simulink model "soccer_vision"  (R2018b)
settings: Solver=FixedStepAuto  StartTime=0.0  StopTime=inf  FixedStep=0.1  RelTol=1e-3
PreLoadFcn:
  | addpath('soccer-vision/media')
  | addpath('soccer-vision/vectormath')
  | 
  | soccer_vision_parameters
InitFcn:
  | soccer_vision_parameters
values from neighbouring files (symbols this model uses):
  imageHeight = 240    [soccer_vision_parameters.m]
  imageWidth = 320    [soccer_vision_parameters.m]
  sampleTime = 1/30    (= 0.0333333333333)    [soccer_vision_parameters.m]
undefined symbols (not defined in the file or in its folder): focal_length, gray, Pose, Rec, SDTV
libraries: robotlib x6, robotcorelib x2, visiontextngfix x2, visiontransforms x2, dspindex x2, simulink_extras x1, visionanalysis x1, visionstatistics x1, visionconversions x1, dspvision x1
settings Model: NumberOfSteps=100  Creator=vuwij  LastModifiedBy=common
settings OptimizationCC: EnhancedBackFolding=on  PassReuseOutputArgsAs=Individual arguments  MaxStackSize=64  OptimizeBlockOrder=speed  DifferentSizesBufferReuse=on  OptimizationCustomize=off
settings DebuggingCC: ParameterTunabilityLossMsg=error  LibraryContextMissingDiagnostic=none
settings HardwareCC: ProdBitPerLong=64  ProdLargestAtomicInteger=Long  ProdLargestAtomicFloat=Double  ProdLongLongMode=on  ProdHWDeviceType=ARM Compatible->ARM 64-bit (LP64)  TargetHWDeviceType=Generic->Unspecified (assume 32-bit Generic)
settings SFSimCC: SimUseLocalCustomCode=off  MATLABDynamicMemAlloc=off
settings RTWCC: SystemTargetFile=ert.tlc  HardwareBoard=Robot Operating System (ROS)  TLCOptions="-aInlineSetEventsForThisBaseRateFcn=TLC_FALSE -aSuppressMultiTaskScheduler=TLC_FALSE  -aRateBasedStepFcn=0"  TemplateMakefile=ert_default_tmf  GenerateReport=on  RTWUseLocalCustomCode=off  Toolchain=Catkin  IncludeHyperlinkInReport=on  LaunchReport=on  PortableWordSizes=on  TargetLang=C++  GenerateTraceInfo=on  GenerateTraceReport=on  GenerateTraceReportSl=on  GenerateTraceReportSf=on  GenerateTraceReportEml=on
settings CodeAppCC: ForceParamTrailComments=on  IgnoreCustomStorageClasses=off  MaxIdLength=95  OperatorAnnotations=on  SimulinkDataObjDesc=on  SFDataObjDesc=on  InsertBlockDesc=on
settings ERTTargetCC: MultiInstanceERTCode=on  CodeInterfacePackaging=C++ class  SupportVariableSizeSignals=on  RootIOFormat=Structure reference

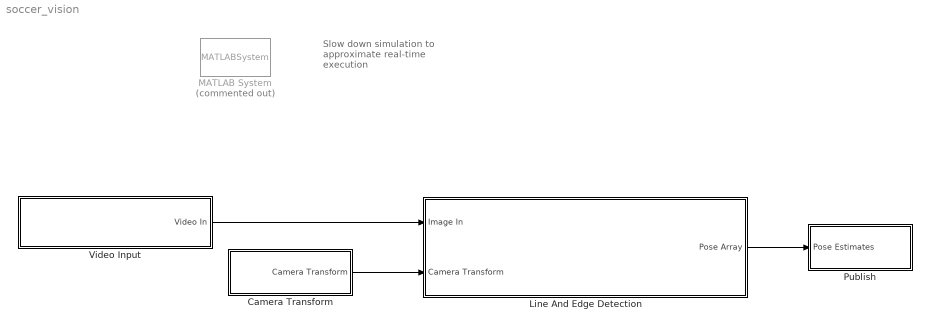
== system soccer_vision ==
  note: Slow down simulation to approximate real-time execution
  Camera Transform : Subsystem  Variant=on
  Line And Edge Detection : Subsystem
  MATLAB System : MATLABSystem  Commented=on  System=ExampleHelperSimulationRateControl  SampleTime=sampleTime
      mask Type: ExampleHelperSimulationRateControl
      mask Display: disp('Rate Control');
  Publish : Subsystem  Variant=on
  Video Input : Subsystem  Variant=on
  wires:
  Video Input/1(Video In) -> Line And Edge Detection/1(Image In)
  Camera Transform/1(Camera Transform) -> Line And Edge Detection/2(Camera Transform)
  Line And Edge Detection/1(Pose Array) -> Publish/1(Pose Estimates)

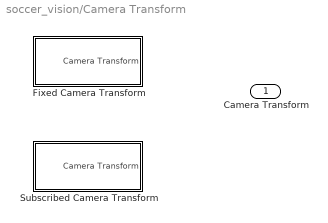
== system soccer_vision/Camera Transform ==
  Fixed Camera Transform : Subsystem  VariantControl=VSS_VIDEO_INPUT
  Subscribed Camera Transform : Subsystem  VariantControl=(default)
  Camera Transform : Outport

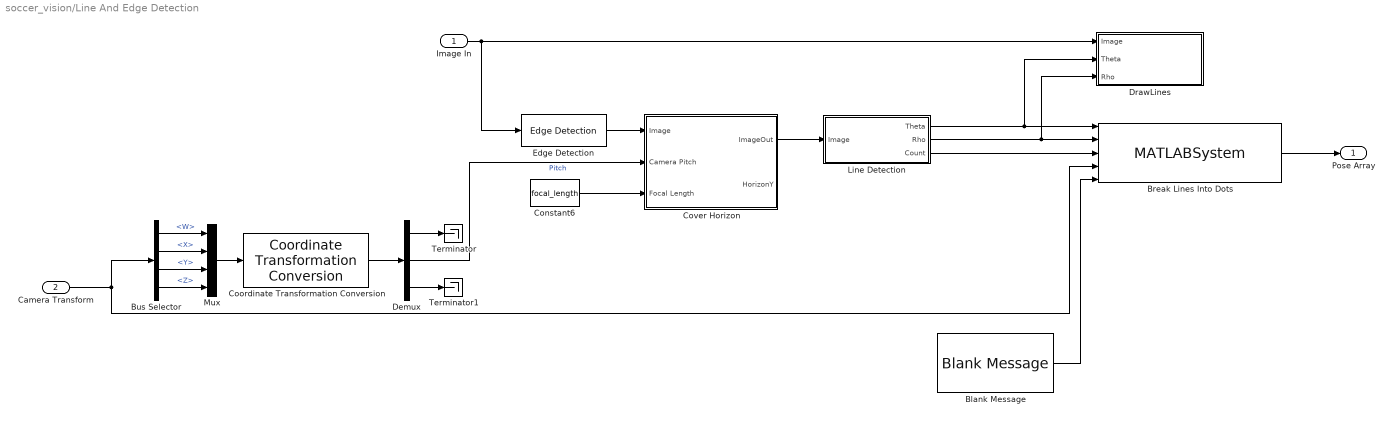
== system soccer_vision/Line And Edge Detection ==
  Image In : Inport  OutDataTypeStr=uint8  PortDimensions=[240 320]  SampleTime=[0.1,0]
  Camera Transform : Inport  Port=2  PortDimensions=1
  Blank Message : robotlib/Blank Message  messageClass=Message  entityType=geometry_msgs/PoseArray  messageType=geometry_msgs/PoseArray  SampleTime=inf
      settings: SourceProductBaseCode=RO
  Break Lines Into Dots : MATLABSystem  System=BreakLinesIntoDots  width=360  height=240  init_pitch=30  init_height=0.5  SimulateUsing=Interpreted execution
      mask Type: BreakLinesIntoDots
      mask Display:
      | disp('BreakLinesIntoDots');
      | port_label('input',1,'thetas');
      | port_label('input',2,'rhos');
      | port_label('input',3,'counts');
      | port_label('input',4,'camerapose');
      | port_label('input',5,'posearray');
      | port_label('output',1,'posearray');
  Bus Selector : BusSelector  OutputSignals=Pose.Orientation.W,Pose.Orientation.X,Pose.Orientation.Y,Pose.Orientation.Z
  Constant6 : Constant  Value=focal_length
  Coordinate Transformation Conversion : robotcorelib/Coordinate Transformation Conversion  InputRepresentation=Quaternion  InputEulerSequence=ZYX  ShowTrVecInputPort=on  OutputRepresentation=Euler Angles  OutputEulerSequence=XYZ  ShowTrVecOutputPort=on  SimulateUsing=Code generation
      settings: SourceProductBaseCode=RO
  Cover Horizon : Subsystem
  Demux : Demux  Outputs=3
  DrawLines : Subsystem
  Edge Detection : visionanalysis/Edge Detection  method=Roberts  outputType=Binary image  userDefinedThreshold=off  thresholdSource=Input port  threshold=20  thresholdTuning=9  edgeThinning=off  threshold_canny=[0.25 0.60]  autoPercent=70  sigma=1  roundingMode=Floor  overflowMode=off  prodOutputMode=Binary point scaling  prodOutputWordLength=32  prodOutputFracLength=8  prodOutputSlope=2^-8  accumSlope=2^-8  outputSlope=2^-4
      settings: SourceProductName=Computer Vision System Toolbox  SourceProductBaseCode=VP
  Line Detection : Subsystem
  Mux : Mux
  Terminator : Terminator
  Terminator1 : Terminator
  Pose Array : Outport
  wires:
  Constant6/1 -> Cover Horizon/3("Focal Length ")
  Demux/2 -> Cover Horizon/2(Camera Pitch)  "Pitch"
  Image In/1 -> Edge Detection/1, DrawLines/1(Image)
  Cover Horizon/1(ImageOut) -> Line Detection/1(Image)
  Edge Detection/1 -> Cover Horizon/1(Image)
  Line Detection/1(Theta) -> DrawLines/2(Theta), Break Lines Into Dots/1
  Line Detection/2(Rho) -> Break Lines Into Dots/2, DrawLines/3(Rho)
  Break Lines Into Dots/1 -> Pose Array/1
  Line Detection/3(Count) -> Break Lines Into Dots/3
  Bus Selector/1 -> Mux/1  "<W>"
  Demux/3 -> Terminator1/1
  Camera Transform/1 -> Break Lines Into Dots/4, Bus Selector/1
  Bus Selector/3 -> Mux/3  "<Y>"
  Demux/1 -> Terminator/1
  Bus Selector/4 -> Mux/4  "<Z>"
  Bus Selector/2 -> Mux/2  "<X>"
  Coordinate Transformation Conversion/1 -> Demux/1
  Mux/1 -> Coordinate Transformation Conversion/1
  Blank Message/1 -> Break Lines Into Dots/5

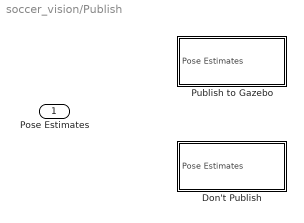
== system soccer_vision/Publish ==
  Pose Estimates : Inport
  Don't Publish : Subsystem  VariantControl=VSS_VIDEO_INPUT
  Publish to Gazebo : Subsystem  VariantControl=(default)

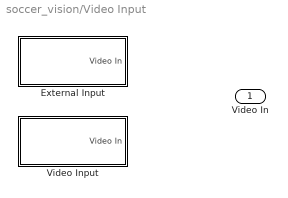
== system soccer_vision/Video Input ==
  External Input : Subsystem  VariantControl=(default)
  Video Input : Subsystem  VariantControl=VSS_VIDEO_INPUT
  Video In : Outport

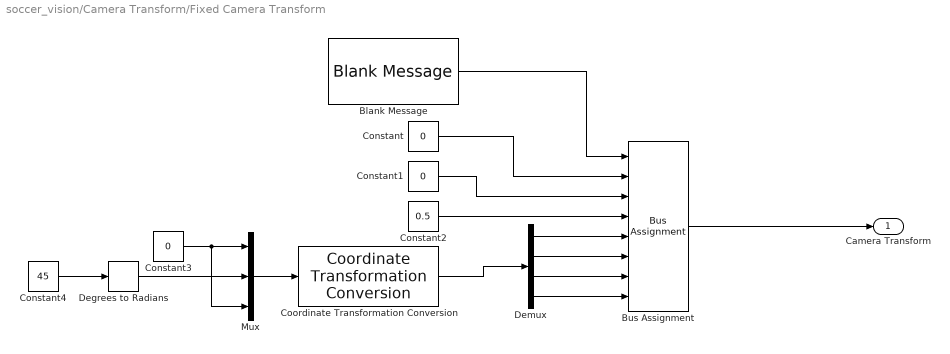
== system soccer_vision/Camera Transform/Fixed Camera Transform ==
  Blank Message : robotlib/Blank Message  messageClass=Message  entityType=geometry_msgs/PoseStamped  messageType=geometry_msgs/PoseStamped  SampleTime=inf
      settings: SourceProductBaseCode=RO
  Bus Assignment : BusAssignment  AssignedSignals=Pose.Position.X,Pose.Position.Y,Pose.Position.Z,Pose.Orientation.X,Pose.Orientation.Y,Pose.Orientation.Z,Pose.Orientation.W
  Constant : Constant  Value=0
  Constant1 : Constant  Value=0
  Constant2 : Constant  Value=0.5
  Constant3 : Constant  Value=0
  Constant4 : Constant  Value=45
  Coordinate Transformation Conversion : robotcorelib/Coordinate Transformation Conversion  InputRepresentation=Euler Angles  InputEulerSequence=ZYX  ShowTrVecInputPort=on  OutputRepresentation=Quaternion  OutputEulerSequence=ZYX  ShowTrVecOutputPort=on  SimulateUsing=Code generation
      settings: SourceProductBaseCode=RO
  Degrees to Radians : simulink_extras/Transformations/Degrees to Radians
  Demux : Demux
  Mux : Mux  Inputs=3
  Camera Transform : Outport
  wires:
  Constant/1 -> Bus Assignment/2
  Blank Message/1 -> Bus Assignment/1
  Bus Assignment/1 -> Camera Transform/1
  Constant1/1 -> Bus Assignment/3
  Constant2/1 -> Bus Assignment/4
  Demux/1 -> Bus Assignment/5
  Demux/2 -> Bus Assignment/6
  Demux/3 -> Bus Assignment/7
  Demux/4 -> Bus Assignment/8
  Coordinate Transformation Conversion/1 -> Demux/1
  Mux/1 -> Coordinate Transformation Conversion/1
  Constant3/1 -> Mux/3, Mux/1
  Degrees to Radians/1 -> Mux/2
  Constant4/1 -> Degrees to Radians/1

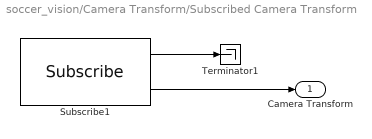
== system soccer_vision/Camera Transform/Subscribed Camera Transform ==
  Subscribe1 : robotlib/Subscribe  topicSource=Specify your own  topic=/soccerbot/poses/camera  messageType=geometry_msgs/Pose  sampleTime=-1  messageQueueLength=1
      settings: SourceProductBaseCode=RO
  Terminator1 : Terminator
  Camera Transform : Outport
  wires:
  Subscribe1/1 -> Terminator1/1
  Subscribe1/2 -> Camera Transform/1

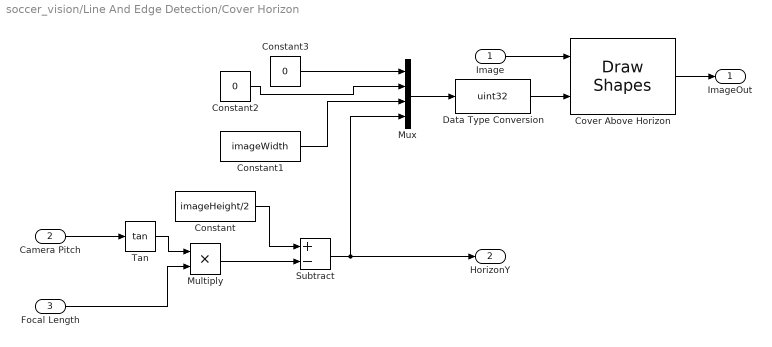
== system soccer_vision/Line And Edge Detection/Cover Horizon ==
  Image : Inport
  Camera Pitch : Inport  Port=2
  "Focal Length " : Inport  Port=3
  Constant : Constant  Value=imageHeight/2
  Constant1 : Constant  Value=imageWidth
  Constant2 : Constant  Value=0
  Constant3 : Constant  Value=0
  Cover Above Horizon : visiontextngfix/Draw Shapes  shape=Rectangles  fill=on  lineWidth=1  fillClrSource=Specify via dialog  display=Black  intensity=200  color=[255 0 0]  opacity=1  viewport=Entire image  antialiasing=off  inType=Obsolete  imagePorts=One multidimensional signal  prodOutputMode=Binary point scaling  prodOutputWordLength=32  prodOutputFracLength=14  memoryMode=Specify word length  memoryWordLength=16  memoryFracLength=14  roundingMode=Floor  overflowMode=off
      settings: SourceProductName=Computer Vision System Toolbox
  Data Type Conversion : DataTypeConversion  OutDataTypeStr=uint32
  Multiply : Product
  Mux : Mux
  Subtract : Sum  Inputs=+-
  Tan : Trigonometry  Operator=tan
  ImageOut : Outport
  HorizonY : Outport  Port=2
  wires:
  Camera Pitch/1 -> Tan/1
  Tan/1 -> Multiply/1
  "Focal Length "/1 -> Multiply/2
  Constant/1 -> Subtract/1
  Multiply/1 -> Subtract/2
  Mux/1 -> Data Type Conversion/1
  Constant3/1 -> Mux/1
  Constant2/1 -> Mux/2
  Constant1/1 -> Mux/3
  Subtract/1 -> Mux/4, HorizonY/1
  Image/1 -> Cover Above Horizon/1
  Data Type Conversion/1 -> Cover Above Horizon/2
  Cover Above Horizon/1 -> ImageOut/1

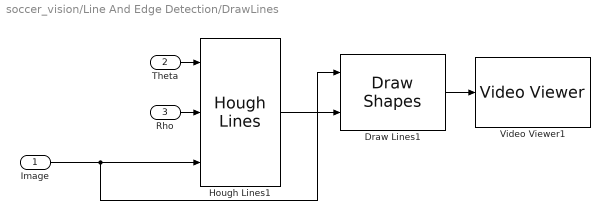
== system soccer_vision/Line And Edge Detection/DrawLines ==
  Image : Inport
  Theta : Inport  Port=2
  Rho : Inport  Port=3
  Draw Lines1 : visiontextngfix/Draw Shapes  shape=Lines  fill=off  lineWidth=1  fillClrSource=Specify via dialog  display=White  intensity=200  color=[255 0 0]  opacity=0.6  viewport=Entire image  antialiasing=off  inType=Obsolete  imagePorts=One multidimensional signal  prodOutputMode=Binary point scaling  prodOutputWordLength=32  prodOutputFracLength=14  memoryMode=Specify word length  memoryWordLength=16  memoryFracLength=14  roundingMode=Floor  overflowMode=off
      settings: SourceProductName=Computer Vision System Toolbox
  Hough Lines1 : visiontransforms/Hough Lines  sineCompMethod=Trigonometric function  thetaRes=pi/180  firstCoeffMode=Specify word length  firstCoeffWordLength=16  firstCoeffFracLength=15  prodOutputMode=Binary point scaling  prodOutputWordLength=32  prodOutputFracLength=16  roundingMode=Nearest  overflowMode=on
      settings: SourceProductName=Computer Vision System Toolbox  SourceProductBaseCode=VP
  Video Viewer1 : VideoViewer  colormapValue=gray(256)  FigPos=[297 924 1134 598]
  wires:
  Theta/1 -> Hough Lines1/1
  Draw Lines1/1 -> Video Viewer1/1
  Hough Lines1/1 -> Draw Lines1/2
  Image/1 -> Draw Lines1/1, Hough Lines1/3
  Rho/1 -> Hough Lines1/2

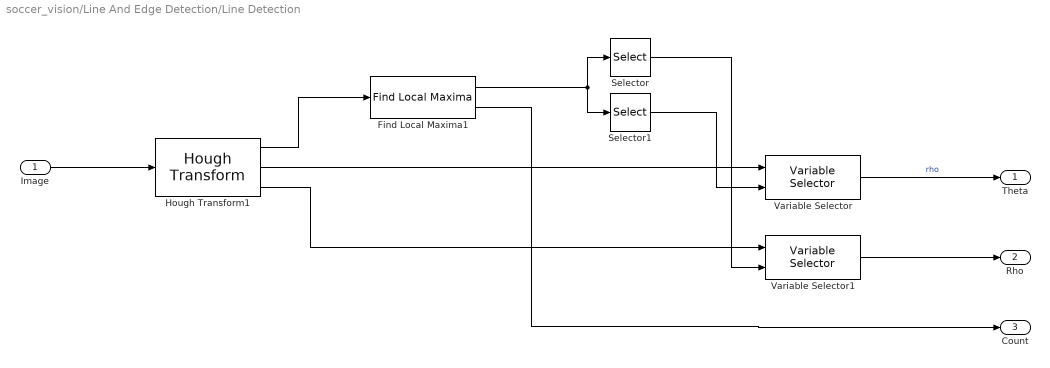
== system soccer_vision/Line And Edge Detection/Line Detection ==
  Image : Inport
  Find Local Maxima1 : visionstatistics/Find Local Maxima  num_peaks=3  nhood_size=[201 41]  src_thresh=Obsolete9b  src_thresh_inuse=Specify via dialog  threshold=100  inputIsHough=on  dt_peak=uint32  isOutVarDim=off  dt_count=uint32
      settings: SourceProductName=Computer Vision System Toolbox  SourceProductBaseCode=VP
  Hough Transform1 : visiontransforms/Hough Transform  theta_res=pi/180  rho_res=1  out_theta_rho=on  outdtmode=double  roundingMode=Nearest  overflowMode=on  firstCoeffMode=Binary point scaling  firstCoeffWordLength=16  firstCoeffFracLength=14  firstCoeffSlope=2^-14  secondCoeffMode=Binary point scaling  secondCoeffWordLength=32  secondCoeffFracLength=16  secondCoeffSlope=2^-16  prodOutputMode=Binary point scaling  prodOutputWordLength=32  prodOutputFracLength=20  prodOutputSlope=2^-20  accumMode=Binary point scaling  accumWordLength=32  accumFracLength=20  accumSlope=2^-20  outputMode=Binary point scaling  outputWordLength=16  outputFracLength=0  outputSlope=2^0  memoryMode=Binary point scaling  memoryWordLength=32  memoryFracLength=16  memorySlope=2^-16
      settings: SourceProductName=Computer Vision System Toolbox  SourceProductBaseCode=VP
  Selector : Selector  NumberOfDimensions=2  InputPortWidth=2  IndexOptions=Select all,Index vector (dialog)  Indices=1,2  OutputSizes=1,1
  Selector1 : Selector  NumberOfDimensions=2  InputPortWidth=2  IndexOptions=Select all,Index vector (dialog)  Indices=0,1  OutputSizes=1,1
  Variable Selector : dspindex/Variable Selector  NumInputs=1  rowsOrCols=Columns  IdxMode=Variable  Elements=[1 3]  ZerOneIdxMode=One-based  errmode=Clip Index  FillMode=on  FillValues=0
  Variable Selector1 : dspindex/Variable Selector  NumInputs=1  rowsOrCols=Columns  IdxMode=Variable  Elements=[1 3]  ZerOneIdxMode=One-based  errmode=Clip Index  FillMode=on  FillValues=0
  Theta : Outport
  Rho : Outport  Port=2
  Count : Outport  Port=3
  wires:
  Hough Transform1/3 -> Variable Selector1/1
  Image/1 -> Hough Transform1/1
  Variable Selector1/1 -> Rho/1
  Variable Selector/1 -> Theta/1  "rho"
  Selector1/1 -> Variable Selector/2
  Selector/1 -> Variable Selector1/2
  Find Local Maxima1/1 -> Selector/1, Selector1/1
  Hough Transform1/2 -> Variable Selector/1
  Hough Transform1/1 -> Find Local Maxima1/1
  Find Local Maxima1/2 -> Count/1

== system soccer_vision/Publish/Don't Publish ==
  Pose Estimates : Inport
  Terminator : Terminator
  wires:
  Pose Estimates/1 -> Terminator/1

== system soccer_vision/Publish/Publish to Gazebo ==
  Pose Estimates : Inport
  Publish : robotlib/Publish  topicSource=Specify your own  topic=/soccerbot/vision_poses  messageType=geometry_msgs/PoseArray  messageQueueLength=1
      settings: SourceProductBaseCode=RO
  wires:
  Pose Estimates/1 -> Publish/1

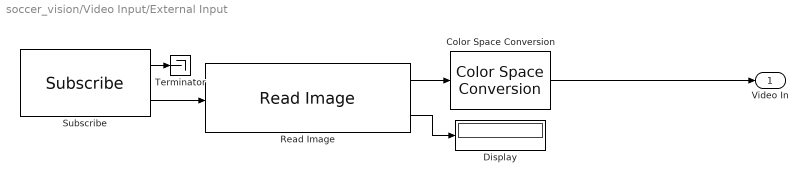
== system soccer_vision/Video Input/External Input ==
  Color Space Conversion : visionconversions/Color Space  Conversion  conversion=Obsolete  conversionActive=R'G'B' to intensity  wp_str=D65  rec=Rec. 601 (SDTV)  sys=1125/60/2:1  imagePorts=One multidimensional signal
      settings: SourceProductName=Computer Vision System Toolbox
  Display : Display
  Read Image : robotlib/Read Image  MaximumImageSize=[240, 320]  ImageEncoding=rgb8  ShowAlphaOutput=off  ShowErrorCodeOutput=on  VariableSizeOutputs=off
      settings: SourceProductName=Robotics System Toolbox  SourceProductBaseCode=RO
  Subscribe : robotlib/Subscribe  topicSource=Select from ROS network  topic=/soccerbot/camera1/image_raw  messageType=sensor_msgs/Image  sampleTime=-1  messageQueueLength=1
      settings: SourceProductBaseCode=RO
  Terminator : Terminator
  Video In : Outport
  wires:
  Color Space Conversion/1 -> Video In/1
  Read Image/1 -> Color Space Conversion/1
  Subscribe/2 -> Read Image/1
  Read Image/2 -> Display/1
  Subscribe/1 -> Terminator/1

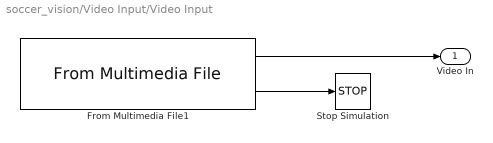
== system soccer_vision/Video Input/Video Input ==
  From Multimedia File1 : dspvision/From Multimedia File  inputFilename=videotestfile  loop=on  numPlays=1  outputStreams=Audio only  videoDataType=uint8  audioDataType=int16  inheritSampleTime=off  userDefinedSampleTime=0.1  noAudioOutput=off  isIntensityVideo=off  fourcc=Intensity  colorVideoFormat=One multidimensional signal  outputEOF=on  dataOrg=Column-major  audioFrameSize=1024  computeAudioFrameSize=off  outSamplingMode=Sample based
      settings: SourceProductBaseCode=VP
  Stop Simulation : Stop
  Video In : Outport
  wires:
  From Multimedia File1/1 -> Video In/1
  From Multimedia File1/2 -> Stop Simulation/1
